simulink model "controller"  (R2024b)
settings: Solver=FixedStepAuto  StartTime=0.0  StopTime=10.0  FixedStep=1/100  RelTol=1e-3
undefined symbols (not defined in the file): MAX_RDB_ENGAGE_SPEED, MAX_SPEED_BACKWARD, MAX_SPEED_FORWARD, MAX_TORQUE, MAX_TORQUE_REVERSE
settings Model: Creator=DAUIN-Win10  LastModifiedBy=feder
settings OptimizationCC: ReuseModelBlockBuffer=off
settings DebuggingCC: UnconnectedInputMsg=warning  UnconnectedOutputMsg=warning  UnconnectedLineMsg=warning
settings ModelReferenceCC: EnableRefExpFcnMdlSchedulingChecks=on
settings RTWCC: GPUComputeCapability=3.5  DLArmComputeVersion=19.05

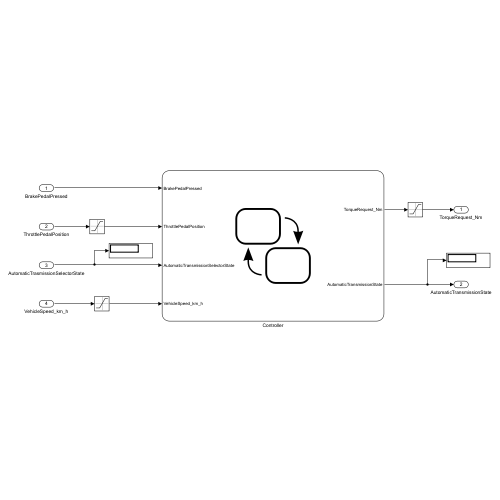
[thumbnail: Simulink's stored preview of the top-level diagram]
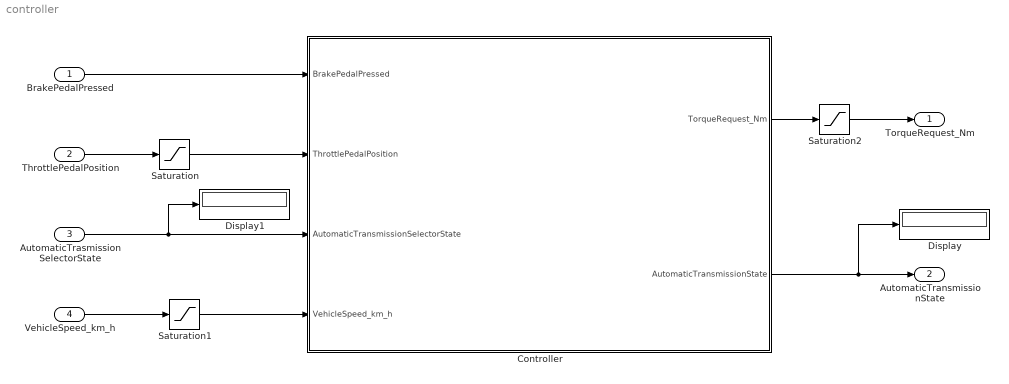
== system controller ==
  BrakePedalPressed : Inport  OutDataTypeStr=boolean
  ThrottlePedalPosition : Inport  Port=2  OutDataTypeStr=single
  AutomaticTrasmissionSelectorState : Inport  Port=3  OutDataTypeStr=Enum: TransmissionState
  VehicleSpeed_km_h : Inport  Port=4  OutDataTypeStr=single  Unit=km/h
  Controller : Stateflow chart  TreatAsAtomicUnit=on
  Display : Display
  Display1 : Display
  Saturation : Saturate  UpperLimit=1  LowerLimit=0
  Saturation1 : Saturate  UpperLimit=MAX_SPEED_FORWARD  LowerLimit=-MAX_SPEED_BACKWARD
  Saturation2 : Saturate  UpperLimit=MAX_TORQUE  LowerLimit=-MAX_TORQUE
  TorqueRequest_Nm : Outport  OutDataTypeStr=single  Unit=N*m
  AutomaticTransmissionState : Outport  Port=2  OutDataTypeStr=Enum: TransmissionState
  wires:
  Controller/2(AutomaticTransmissionState) -> Display/1, AutomaticTransmissionState/1
  AutomaticTrasmissionSelectorState/1 -> Display1/1, Controller/3(AutomaticTransmissionSelectorState)
  ThrottlePedalPosition/1 -> Saturation/1
  Saturation/1 -> Controller/2(ThrottlePedalPosition)
  VehicleSpeed_km_h/1 -> Saturation1/1
  Saturation1/1 -> Controller/4(VehicleSpeed_km_h)
  BrakePedalPressed/1 -> Controller/1(BrakePedalPressed)
  Controller/1(TorqueRequest_Nm) -> Saturation2/1
  Saturation2/1 -> TorqueRequest_Nm/1

== stateflow chart controller/Controller ==
  state Park
    entry:
    AutomaticTransmissionState = TransmissionState.Park;
    during:
    TorqueRequest_Nm = 0;
  state Reverse
    entry:
    AutomaticTransmissionState = TransmissionState.Reverse;
    during:
    state BackwardAcceleration
      during:
      TorqueRequest_Nm = -MAX_TORQUE_REVERSE*ThrottlePedalPosition;
    state BackwardRestart
      during:
      TorqueRequest_Nm = -MAX_TORQUE_REVERSE/20;
    state Stop
      during:
      TorqueRequest_Nm = 0;
    (default) -> BackwardAcceleration
    BackwardRestart -> BackwardAcceleration : [BrakePedalPressed == 0 && ThrottlePedalPosition > 0]
    BackwardAcceleration -> Reverse.Stop : [BrakePedalPressed == 1]
    Reverse.Stop -> BackwardAcceleration [order 2] : [BrakePedalPressed == 0]
    (junction 77) -> BackwardRestart
    Reverse.Stop -> (junction 77) [order 1] : [BrakePedalPressed == 0 && abs(VehicleSpeed_km_h) <= MAX_RDB_ENGAGE_SPEED]
  state Brake
    entry:
    AutomaticTransmissionState = TransmissionState.Brake;
    state Acceleration
      during:
      TorqueRequest_Nm = MAX_TORQUE*3/2*(ThrottlePedalPosition-1/3);
    state Restart
      during:
      TorqueRequest_Nm = MAX_TORQUE/20;
    state EmergencyStop
      during:
      TorqueRequest_Nm = 0;
    state Stop
      during:
      TorqueRequest_Nm = 0;
    state RegenarativeBraking
      during:
      TorqueRequest_Nm = -MAX_TORQUE*(1-3*ThrottlePedalPosition);
    (default) -> Brake.Acceleration
    Brake.Restart -> Brake.Acceleration [order 2] : [VehicleSpeed_km_h > MAX_RDB_ENGAGE_SPEED]
    Brake.Acceleration -> (junction 123) [order 2] : [BrakePedalPressed == 1]
    (junction 123) -> EmergencyStop
    Brake.Acceleration -> RegenarativeBraking [order 1] : [ThrottlePedalPosition <= 1/3]
    RegenarativeBraking -> Brake.Acceleration [order 1] : [ThrottlePedalPosition > 1/3]
    Brake.Restart -> Brake.Stop [order 1] : [ThrottlePedalPosition <= 1/3 || BrakePedalPressed ==1]
    Brake.Stop -> Brake.Restart [order 1] : [ThrottlePedalPosition > 1/3]
    EmergencyStop -> (junction 127) : [BrakePedalPressed == 0]
    (junction 127) -> RegenarativeBraking
    (junction 134) -> EmergencyStop
    (junction 190) -> EmergencyStop
    RegenarativeBraking -> (junction 134) [order 3] : [BrakePedalPressed == 1]
    Brake.Stop -> (junction 190) [order 2] : [BrakePedalPressed == 1]
    RegenarativeBraking -> Brake.Stop [order 2] : [VehicleSpeed_km_h <= MAX_RDB_ENGAGE_SPEED]
  state Drive
    entry:
    AutomaticTransmissionState = TransmissionState.Drive;
    state Acceleration
      during:
      TorqueRequest_Nm = MAX_TORQUE*ThrottlePedalPosition;
    state Restart
      during:
      TorqueRequest_Nm = MAX_TORQUE/20;
    state Stop
      during:
      TorqueRequest_Nm = 0;
    (default) -> Drive.Acceleration
    Drive.Restart -> Drive.Acceleration : [BrakePedalPressed == 0 && ThrottlePedalPosition > 0]
    Drive.Acceleration -> Drive.Stop : [BrakePedalPressed == 1]
    Drive.Stop -> Drive.Acceleration [order 2] : [BrakePedalPressed == 0]
    (junction 62) -> Drive.Restart
    Drive.Stop -> (junction 62) [order 1] : [BrakePedalPressed == 0 && VehicleSpeed_km_h <= MAX_RDB_ENGAGE_SPEED]
  state Neutral
    entry:
    AutomaticTransmissionState = TransmissionState.Neutral;
    during:
    TorqueRequest_Nm = 0;
  (default) -> Park
  Neutral -> Park [order 3] : [abs(VehicleSpeed_km_h) < 5 && BrakePedalPressed == 1 && AutomaticTransmissionSelectorState == 0]
  Park -> Neutral : [BrakePedalPressed == 1 && AutomaticTransmissionSelectorState ~= 0]
  Brake -> Drive : [AutomaticTransmissionSelectorState ~= 4]
  Drive -> Neutral [order 1] : [AutomaticTransmissionSelectorState == 0 || AutomaticTransmissionSelectorState == 1 || AutomaticTransmissionSelectorState == 2]
  Neutral -> Reverse [order 2] : [VehicleSpeed_km_h < 5 && BrakePedalPressed == 1 && AutomaticTransmissionSelectorState == 1]
  Reverse -> Neutral : [AutomaticTransmissionSelectorState ~= 1]
  Neutral -> Drive [order 1] : [VehicleSpeed_km_h > -5 && BrakePedalPressed == 1 && (AutomaticTransmissionSelectorState == 4|| AutomaticTransmissionSelectorState == 3) ]
  Drive -> Brake [order 2] : [ThrottlePedalPosition > 1/3 && AutomaticTransmissionSelectorState == 4]
  data: BrakePedalPressed input boolean; ThrottlePedalPosition input single; AutomaticTransmissionSelectorState input Enum: TransmissionState; MAX_TORQUE parameter single; MAX_RDB_ENGAGE_SPEED parameter single; TorqueRequest_Nm output single; AutomaticTransmissionState output Enum: TransmissionState; VehicleSpeed_km_h input single; MAX_TORQUE_REVERSE parameter single
